simulink model "anc2_fxlms"  (R2013a)
settings: Solver=VariableStepDiscrete  StartTime=0.0  StopTime=0.5  RelTol=1e-3
libraries: simulink x1
settings Model: Creator=balazs.varga  LastModifiedBy=balazs.varga

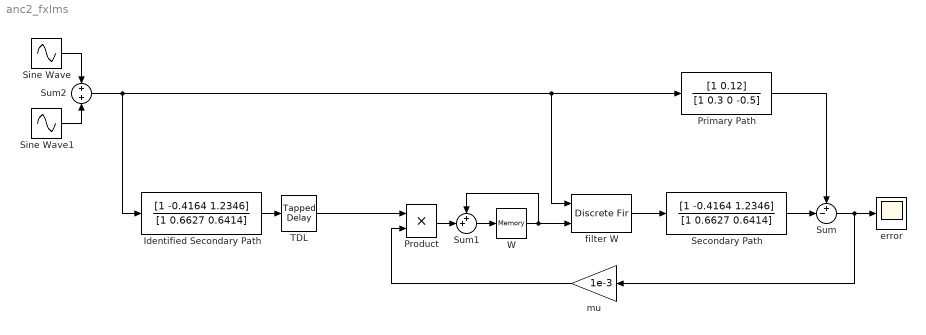
== system anc2_fxlms ==
  Identified Secondary Path : DiscreteFilter  Numerator=[1 -0.4164 1.2346]  Denominator=[1 0.6627 0.6414]  SampleTime=1/8000
  Primary Path : DiscreteFilter  Numerator=[1 0.12]  Denominator=[1 0.3 0 -0.5]  SampleTime=1/8000
  Product : Product  SampleTime=1/8000
  Secondary Path : DiscreteFilter  Numerator=[1 -0.4164 1.2346]  Denominator=[1 0.6627 0.6414]  SampleTime=1/8000
  Sine Wave : Sin  Frequency=2*pi*440  SampleTime=0
  Sine Wave1 : Sin  Amplitude=2  Frequency=2*pi*sqrt(3)*440  SampleTime=0
  Sum : Sum  Inputs=+-|  SampleTime=1/8000
  Sum1 : Sum  Inputs=++|  SampleTime=1/8000
  Sum2 : Sum  Inputs=+|+  SampleTime=1/8000
  TDL : simulink/Discrete/Tapped Delay  vinit=0.0  samptime=1/8000  NumDelays=99  DelayOrder=Newest  includeCurrent=on
  W : Memory  X0=zeros(1,100)  InheritSampleTime=on
  error : Scope
      settings: YMin=-0.3  YMax=0.45
  filter W : DiscreteFir  CoefSource=Input port  SampleTime=1/8000
  mu : Gain  Gain=1e-3  SampleTime=1/8000
  wires:
  W/1 -> filter W/2, Sum1/1
  Sum/1 -> mu/1, error/1
  Sum1/1 -> W/1
  Product/1 -> Sum1/2
  Primary Path/1 -> Sum/1
  Secondary Path/1 -> Sum/2
  filter W/1 -> Secondary Path/1
  Sum2/1 -> Identified Secondary Path/1, filter W/1, Primary Path/1
  Identified Secondary Path/1 -> TDL/1
  TDL/1 -> Product/1
  Sine Wave/1 -> Sum2/1
  Sine Wave1/1 -> Sum2/2
  mu/1 -> Product/2
